simulink model "svpwm_test"  (R2016a)
settings: Solver=VariableStepAuto  StartTime=0.0  StopTime=10.0  RelTol=1e-3
settings Model: Creator=LRF  LastModifiedBy=LRF

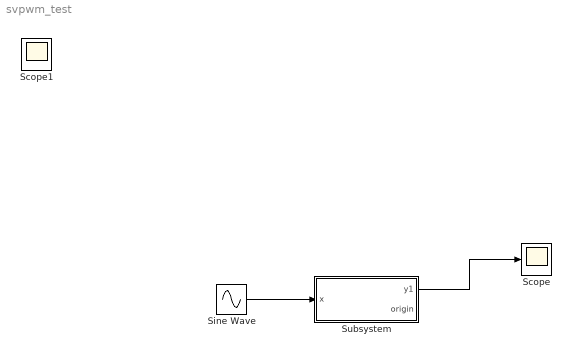
== system svpwm_test ==
  Scope : Scope
  Sine Wave : Sin  SampleTime=0
  Subsystem : Subsystem  mask{m=5, n=2}
      mask prompts: m "Gain"; n "Constant"
      mask init:
      | t=[0:0.05:1];
      | y1=sin(2*pi*t);
      | y2=m*sin(2*pi*t)+n;
      mask Display:
      | plot(t,y1);
      | plot(t,y2);
  Scope1 : Scope
  wires:
  Sine Wave/1 -> Subsystem/1(x)
  Subsystem/1(y1) -> Scope/1

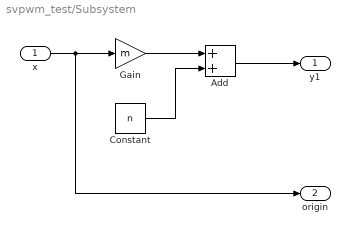
== system svpwm_test/Subsystem ==
  x : Inport
  Add : Sum
  Constant : Constant  Value=n
  Gain : Gain  Gain=m
  y1 : Outport
  origin : Outport  Port=2
  wires:
  x/1 -> origin/1, Gain/1
  Gain/1 -> Add/1
  Constant/1 -> Add/2
  Add/1 -> y1/1
